simulink model "current_controller_post_process"  (R2025b)
settings: Solver=VariableStepAuto  StartTime=0.0  StopTime=2  RelTol=1e-3  EnableMultiTasking=on
InitFcn:
  | ts = prepareLogForParameterEstimation("../LOGS/log0168.csv")
settings Model: ModifiedByFormat=The MathWorks Inc.  Creator=The MathWorks, Inc.  LastModifiedBy=The MathWorks Inc.
settings SolverCC: AlgebraicLoopSolver=TrustRegion  AutoInsertRateTranBlk=on
settings DataIOCC: LimitDataPoints=on  SaveFormat=Array  SaveOutput=off  SaveTime=off  ReturnWorkspaceOutputs=off
settings OptimizationCC: DefaultUnderspecifiedDataType=single  ExpressionDepthLimit=2147483647.0  LifeSpan=1
settings DebuggingCC: UnderspecifiedInitializationDetection=Classic  MergeDetectMultiDrivingBlocksExec=none  SolverPrmCheckMsg=warning  FcnCallInpInsideContextMsg=warning  UnconnectedInputMsg=warning  UnconnectedOutputMsg=warning  UnconnectedLineMsg=warning  StateNameClashWarn=warning  SFUnexpectedBacktrackingDiag=warning  SFNoUnconditionalDefaultTransitionDiag=warning  SFExecutionAtInitializationDiag=none  ArithmeticOperatorsInVariantConditions=warning
settings HardwareCC: ProdBitPerPointer=32.0  ProdBitPerSizeT=32.0  ProdBitPerPtrDiffT=32.0  ProdLargestAtomicFloat=None  ProdIntDivRoundTo=Undefined  ProdEndianess=Unspecified  ProdWordSize=32.0  ProdHWDeviceType=32-bit Generic
settings ModelReferenceCC: PropagateSignalLabelsOutOfModel=off
settings SFSimCC: SimUseLocalCustomCode=off  CustomCodeUndefinedFunction=UseInterfaceOnly
settings RTWCC: RTWUseLocalCustomCode=off  GPUComputeCapability=3.5
settings CodeAppCC: StateflowObjectComments=on
settings GRTTargetCC: TargetLangStandard=C89/C90 (ANSI)  CombineOutputUpdateFcns=off  GRTInterface=on
settings ConfigComp: CovMetricSettings=dw  CovSaveCumulativeToWorkspaceVar=on  CovSaveSingleToWorkspaceVar=on  CovExternalEMLEnable=off  CovSFcnEnable=off

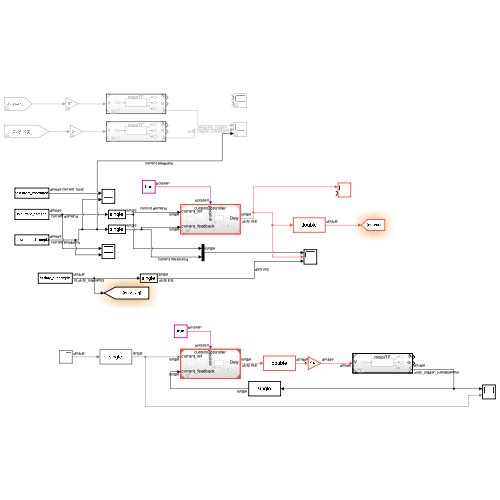
[thumbnail: Simulink's stored preview of the top-level diagram]
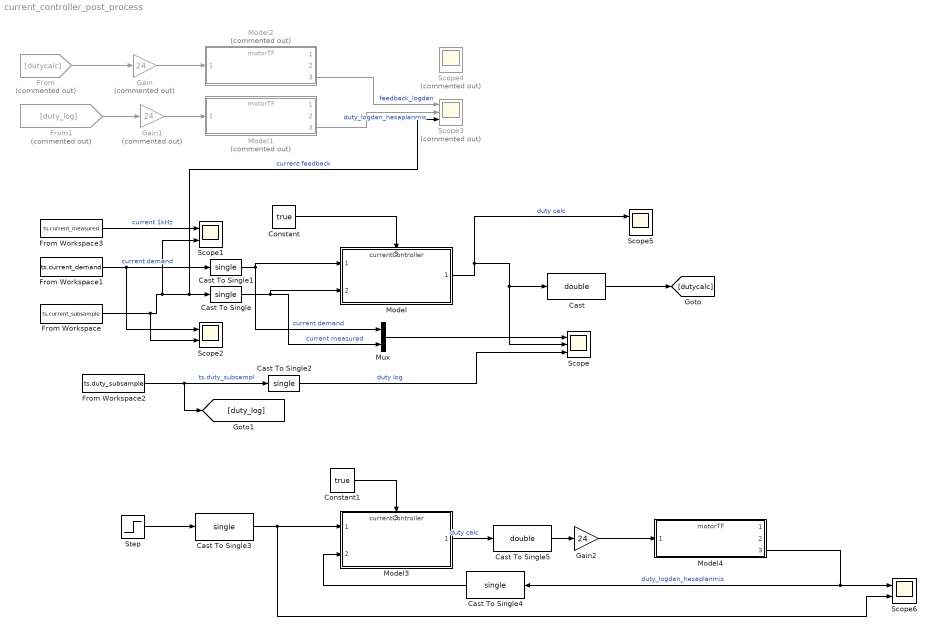
== system current_controller_post_process ==
  Cast : DataTypeConversion  OutDataTypeStr=double  SaturateOnIntegerOverflow=off  RndMeth=Floor
  Cast To Single{,1..4} (5 alike) : DataTypeConversion  OutDataTypeStr=single  SaturateOnIntegerOverflow=off  RndMeth=Floor
  Cast To Single5 : DataTypeConversion  OutDataTypeStr=double  SaturateOnIntegerOverflow=off  RndMeth=Floor
  Constant : Constant  Value=true
  Constant1 : Constant  Value=true
  From : From  Commented=on  GotoTag=dutycalc
  From Workspace : FromWorkspace  VariableName=ts.current_subsample  Interpolate=off  OutputAfterFinalValue=Holding final value
  From Workspace1 : FromWorkspace  VariableName=ts.current_demand  Interpolate=off  OutputAfterFinalValue=Holding final value
  From Workspace2 : FromWorkspace  VariableName=ts.duty_subsample  SampleTime=-1  Interpolate=off  OutputAfterFinalValue=Holding final value
  From Workspace3 : FromWorkspace  VariableName=ts.current_measured  Interpolate=off  OutputAfterFinalValue=Holding final value
  From1 : From  Commented=on  GotoTag=duty_log
  Gain : Gain  Commented=on  Gain=24
  Gain1 : Gain  Commented=on  Gain=24
  Gain2 : Gain  Gain=24
  Model : ModelReference  ModelNameDialog=currentController.slx  SimulationMode=Normal  ModelReferenceVersion=1.63
      settings: PortSchema="{\"entries\":[{\"content\":{\"sides\":[{\"content\":{\"connectorIds\":[\"In1\",\"In2\"]},\"type\":\"ConnectorPlacement.EquallySpacedRectSide\",\"uuid\":\"23f1008d-9fb4-43a2-9c32-1e5e859d66b6\"},{\"content\":{\"connectorIds\":[\"Out1\"],\"side\":\"RIGHT\"},\"type\":\"ConnectorPlacement.EquallySpacedRectSide\",\"uuid\":\"5f1840ba-6133-4c96-bb41-065a993846ec\"},{\"content\":{\"connectorIds\":[\"In3\"],\"side\":\"TOP\"},\"type\":\"ConnectorPlacement.EquallySpacedRectSide\",\"uuid\":\"32bb69cd-874d-46b5-9a8b-12c9b1e0711c\"}]},\"type\":\"ConnectorPlacement.EquallySpacedConnector\",\"uuid\":\"255c90ee-c6ac-4977-a8dd-9220994fed7e\"}],\"packageUris\":[\"http://schema.mathworks.com/mf0/Connector/R2020b\"],\"version\":\"1.0\"}"
  Model1 : ModelReference  Commented=on  ModelNameDialog=motorTF.slx  SimulationMode=Normal  ModelReferenceVersion=1.3
  Model2 : ModelReference  Commented=on  ModelNameDialog=motorTF.slx  SimulationMode=Normal  ModelReferenceVersion=1.3
  Model3 : ModelReference  ModelNameDialog=currentController.slx  SimulationMode=Normal  ModelReferenceVersion=1.63
      settings: PortSchema="{\"entries\":[{\"content\":{\"sides\":[{\"content\":{\"connectorIds\":[\"In1\",\"In2\"]},\"type\":\"ConnectorPlacement.EquallySpacedRectSide\",\"uuid\":\"23f1008d-9fb4-43a2-9c32-1e5e859d66b6\"},{\"content\":{\"connectorIds\":[\"Out1\"],\"side\":\"RIGHT\"},\"type\":\"ConnectorPlacement.EquallySpacedRectSide\",\"uuid\":\"5f1840ba-6133-4c96-bb41-065a993846ec\"},{\"content\":{\"connectorIds\":[\"In3\"],\"side\":\"TOP\"},\"type\":\"ConnectorPlacement.EquallySpacedRectSide\",\"uuid\":\"32bb69cd-874d-46b5-9a8b-12c9b1e0711c\"}]},\"type\":\"ConnectorPlacement.EquallySpacedConnector\",\"uuid\":\"255c90ee-c6ac-4977-a8dd-9220994fed7e\"}],\"packageUris\":[\"http://schema.mathworks.com/mf0/Connector/R2020b\"],\"version\":\"1.0\"}"
  Model4 : ModelReference  ModelNameDialog=motorTF.slx  SimulationMode=Normal  ModelReferenceVersion=1.3
  Mux : Mux  Inputs=2
  Scope : Scope  NumInputPorts=3
      settings: ActiveDisplayYMinimum=-14.668013453483582  ActiveDisplayYMaximum=18.52390468120575
  Scope{1..2,5..6} (4 alike) : Scope  NumInputPorts=2
      Scope1 settings: ActiveDisplayYMinimum=-0.43060109158977866  ActiveDisplayYMaximum=0.0358955687843263
      Scope2 settings: ActiveDisplayYMinimum=-14.668013453483582  ActiveDisplayYMaximum=18.52390468120575  DataLoggingVariableName=ScopeData2
      Scope5 settings: ActiveDisplayYMinimum=-40.032722353935235  ActiveDisplayYMaximum=230.13589560985565  DataLoggingVariableName=ScopeData5
      Scope6 settings: ActiveDisplayYMinimum=0.48865477402148982  ActiveDisplayYMaximum=0.49134154341346936  DataLoggingVariableName=ScopeData6
  Scope3 : Scope  Commented=on  NumInputPorts=3
      settings: ActiveDisplayYMinimum=-15.134162039668784  ActiveDisplayYMaximum=18.57569896855966  DataLoggingVariableName=ScopeData3
  Scope4 : Scope  Commented=on  NumInputPorts=2
      settings: ActiveDisplayYMinimum=-0.58156470171662811  ActiveDisplayYMaximum=0.38877860289161387  DataLoggingVariableName=ScopeData4
  Step : Step  After=0.5  SampleTime=0
  wires:
  From Workspace1/1 -> Cast To Single1/1, Scope2/1  "current demand"
  From Workspace/1 -> Scope1/2, Scope3/3, Cast To Single/1, Scope2/2  "current feedback"
  Mux/1 -> Scope/1
  Cast To Single/1 -> Model/2, Mux/2  "current measured"
  Cast To Single1/1 -> Model/1, Mux/1  "current demand"
  From Workspace2/1 -> Cast To Single2/1, [duty_log]  "ts.duty_subsampl"
  Cast To Single2/1 -> Scope/3  "duty log"
  From Workspace3/1 -> Scope1/1  "current 1kHz"
  Constant/1 -> Model/3
  Model/1 -> Scope5/1, Scope/2, Cast/1  "duty calc"
  From/1 -> Gain/1
  From1/1 -> Gain1/1
  Model2/3 -> Scope3/1  "feedback_logdan"
  Model1/3 -> Scope3/2  "duty_logdan_hesaplanmis"
  Cast/1 -> [dutycalc]
  Gain/1 -> Model2/1
  Gain1/1 -> Model1/1
  Step/1 -> Cast To Single3/1
  Model3/1 -> Cast To Single5/1  "duty calc"
  Constant1/1 -> Model3/3
  Model4/3 -> Cast To Single4/1, Scope6/1  "duty_logdan_hesaplanmis"
  Cast To Single3/1 -> Scope6/2, Model3/1
  Cast To Single4/1 -> Model3/2
  Cast To Single5/1 -> Gain2/1
  Gain2/1 -> Model4/1
